simulink model "ninelevelCHBinverter"  (R2023a)
settings: Solver=VariableStepAuto  StartTime=0.0  StopTime=0.1  RelTol=1e-3
libraries: spsIGBTDiodeLib x16, simulink x8, spsDCVoltageSourceLib x4, spsVoltageMeasurementLib x1, sps_lib x1
settings Model: Creator=User  LastModifiedBy=User

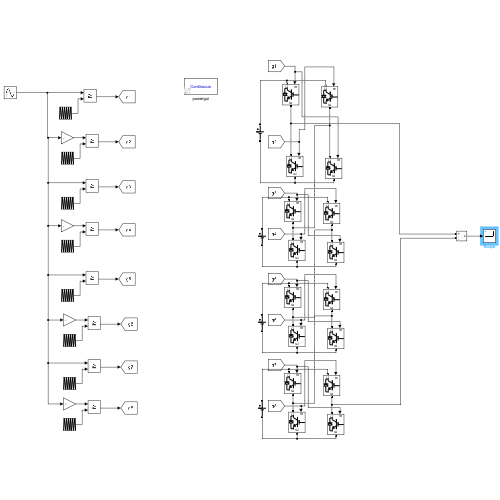
[thumbnail: Simulink's stored preview of the top-level diagram]
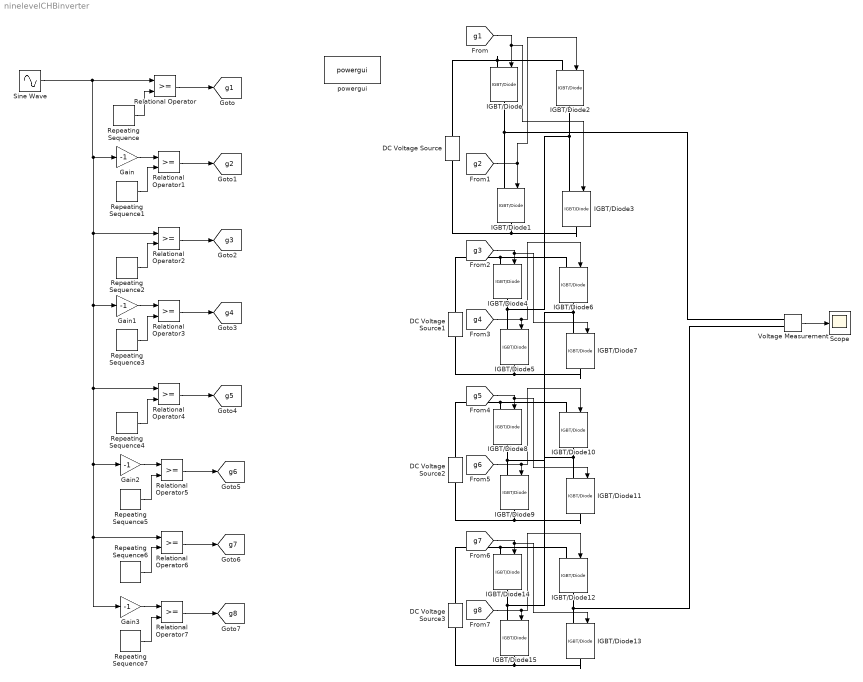
== system ninelevelCHBinverter ==
  DC Voltage Source{,1..3} (4 alike) : spsDCVoltageSourceLib/DC Voltage Source  Amplitude=100  Measurements=None
  Gain{,1..3} (4 alike) : Gain  Gain=-1
  IGBT/Diode{,1..15} (16 alike) : spsIGBTDiodeLib/IGBT//Diode  Ron=1e-3  Rs=1e5  Cs=inf  Measurements=off
  Relational Operator{,1..7} (8 alike) : RelationalOperator  OutDataTypeStr=boolean  RndMeth=Simplest  InputSameDT=off
  Repeating Sequence : simulink/Sources/Repeating Sequence  rep_seq_t=[0 1 2 3 4]*0.001*0.5  rep_seq_y=[0 1 0 1 0]
  Repeating Sequence1 : simulink/Sources/Repeating Sequence  rep_seq_t=[0 1 2 3 4]*0.001*0.5  rep_seq_y=[0 1 0 1 0]
  Repeating Sequence2 : simulink/Sources/Repeating Sequence  rep_seq_t=[0 1 2 3 4]*0.001*0.5  rep_seq_y=[1 2 1 2 1]
  Repeating Sequence3 : simulink/Sources/Repeating Sequence  rep_seq_t=[0 1 2 3 4]*0.001*0.5  rep_seq_y=[1 2 1 2 1]
  Repeating Sequence4 : simulink/Sources/Repeating Sequence  rep_seq_t=[0 1 2 3 4]*0.001*0.5  rep_seq_y=[2 3 2 3 2]
  Repeating Sequence5 : simulink/Sources/Repeating Sequence  rep_seq_t=[0 1 2 3 4]*0.001*0.5  rep_seq_y=[2 3 2 3 2]
  Repeating Sequence6 : simulink/Sources/Repeating Sequence  rep_seq_t=[0 1 2 3 4]*0.001*0.5  rep_seq_y=[3 4 3 4 3]
  Repeating Sequence7 : simulink/Sources/Repeating Sequence  rep_seq_t=[0 1 2 3 4]*0.001*0.5  rep_seq_y=[3 4 3 4 3]
  Scope : Scope
  Sine Wave : Sin  Amplitude=4  Frequency=2*pi*50  SampleTime=0
  Voltage Measurement : spsVoltageMeasurementLib/Voltage Measurement  PhasorSimulation=off  OutputType=Complex  PSBequivalent=0
  powergui : sps_lib/powergui  Priority=1  SimulationMode=Continuous  SampleTime=50e-6  frequency=60  Iterations=50  frequencyindice=0  Pbase=100e6  ErrMax=1e-4  UnitsV=kV  UnitsW=MW  buscounter=0  FunctionMessages=off  echomessages=off  EnableUseOfTLC=off  CurrentSourceSwitches=off  DisableSnubberDevices=off  DisableRonSwitches=off  DisableVfSwitches=off  DisplayEquations=off  AutomaticDiscreteSolvers=off  SolverType=Tustin/Backward Euler (TBE)  Interpol=off  ExternalGateDelay=off  methode=off  Ts=100  x0status=blocks  SPID=on  SwTol=0  HookPort=off  NonlinearTolerance=1e-4  nMaxIteration=100  ContinueOnMaxIteration=off  RestoreLinks=warning  ResistiveCurrentMeasurement=off  Frange=[0:2:500]  Ylog=off  Xlog=on  ShowGrid=off  save=off  variable=ZData  structure=0  ZoomFFT=off  StartTime=0.0  cycles=1  DisplayStyle=1  fundamental=60  FreqAxis=off  MaxFrequency=1000  frequencyindicesteady=1  RmsSteady=1  display=off
  tag scope: g1=global, g2=global, g3=global, g4=global, g5=global, g6=global, g7=global, g8=global
  wires:
  Relational Operator5/1 -> [g6]
  [g6] -> IGBT/Diode10/1, IGBT/Diode9/1
  Repeating Sequence4/1 -> Relational Operator4/2
  Relational Operator/1 -> [g1]
  [g1] -> IGBT/Diode3/1, IGBT/Diode/1
  Repeating Sequence1/1 -> Relational Operator1/2
  [g2] -> IGBT/Diode2/1, IGBT/Diode1/1
  [g4] -> IGBT/Diode6/1, IGBT/Diode5/1
  Repeating Sequence3/1 -> Relational Operator3/2
  [g3] -> IGBT/Diode7/1, IGBT/Diode4/1
  Relational Operator4/1 -> [g5]
  Repeating Sequence2/1 -> Relational Operator2/2
  Relational Operator1/1 -> [g2]
  Repeating Sequence5/1 -> Relational Operator5/2
  Relational Operator2/1 -> [g3]
  [g5] -> IGBT/Diode11/1, IGBT/Diode8/1
  Relational Operator3/1 -> [g4]
  Voltage Measurement/1 -> Scope/1
  Repeating Sequence/1 -> Relational Operator/2
  [g7] -> IGBT/Diode13/1, IGBT/Diode14/1
  [g8] -> IGBT/Diode12/1, IGBT/Diode15/1
  Relational Operator6/1 -> [g7]
  Repeating Sequence6/1 -> Relational Operator6/2
  Relational Operator7/1 -> [g8]
  Sine Wave/1 -> Gain/1, Gain1/1, Gain2/1, Gain3/1, Relational Operator6/1, Relational Operator4/1, Relational Operator2/1, Relational Operator/1
  Repeating Sequence7/1 -> Relational Operator7/2
  Gain/1 -> Relational Operator1/1
  Gain1/1 -> Relational Operator3/1
  Gain2/1 -> Relational Operator5/1
  Gain3/1 -> Relational Operator7/1
  connections:
  DC Voltage Source2/RConn1 -- IGBT/Diode8/LConn1 -- IGBT/Diode10/LConn1
  IGBT/Diode14/RConn1 -- IGBT/Diode10/RConn1 -- IGBT/Diode11/LConn1 -- IGBT/Diode15/LConn1
  DC Voltage Source1/RConn1 -- IGBT/Diode4/LConn1 -- IGBT/Diode6/LConn1
  IGBT/Diode/LConn1 -- IGBT/Diode2/LConn1 -- DC Voltage Source/RConn1
  IGBT/Diode1/LConn1 -- Voltage Measurement/LConn1 -- IGBT/Diode/RConn1
  IGBT/Diode2/RConn1 -- IGBT/Diode3/LConn1 -- IGBT/Diode5/LConn1 -- IGBT/Diode4/RConn1
  IGBT/Diode1/RConn1 -- IGBT/Diode3/RConn1 -- DC Voltage Source/LConn1
  DC Voltage Source2/LConn1 -- IGBT/Diode9/RConn1 -- IGBT/Diode11/RConn1
  DC Voltage Source1/LConn1 -- IGBT/Diode5/RConn1 -- IGBT/Diode7/RConn1
  IGBT/Diode7/LConn1 -- IGBT/Diode9/LConn1 -- IGBT/Diode8/RConn1 -- IGBT/Diode6/RConn1
  DC Voltage Source3/LConn1 -- IGBT/Diode15/RConn1 -- IGBT/Diode13/RConn1
  DC Voltage Source3/RConn1 -- IGBT/Diode14/LConn1 -- IGBT/Diode12/LConn1
  IGBT/Diode13/LConn1 -- Voltage Measurement/LConn2 -- IGBT/Diode12/RConn1
